simulink model "blackbanana_kinlam_ver2"  (R2022b)
settings: Solver=VariableStepAuto  StartTime=0.0  StopTime=20  RelTol=1e-3
model workspace: external: MAT-File params.mat (data not in the file)
undefined symbols (not defined in the file): cache_size, fleet_size, lambda_allocated_memory, lambda_parallel_instances, message_size, simulation_time, time
libraries: simulink x2, VACLib x1
settings Model: Creator=KarlO  LastModifiedBy=KarlO

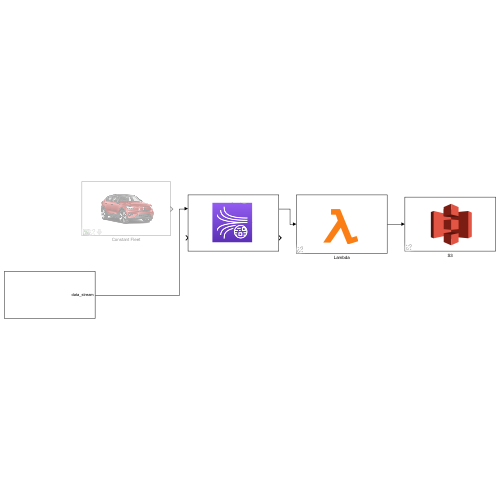
[thumbnail: Simulink's stored preview of the top-level diagram]
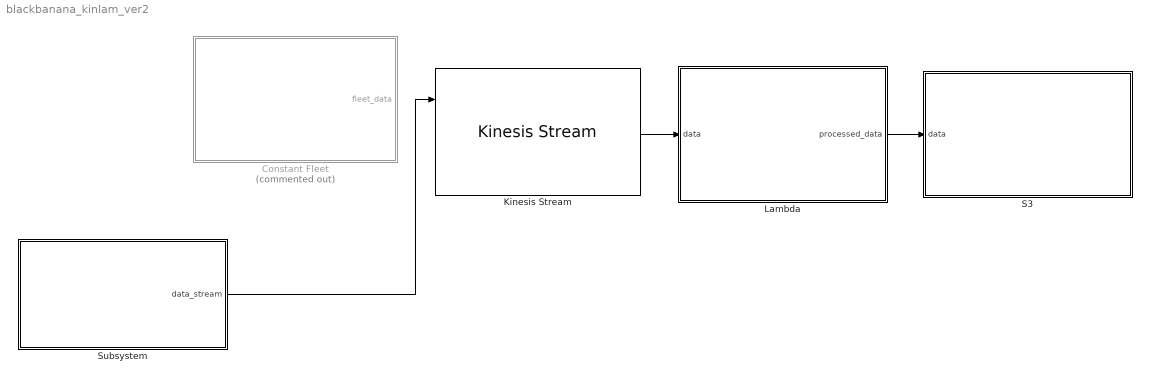
== system blackbanana_kinlam_ver2 ==
  Constant Fleet : Subsystem  Commented=on  AncestorBlock=VACLib/Vehicle Components/Constant Fleet  mask{fleet_size=0, cache_size=0, simulation_time=0, message_size=0}
      settings: LibrarySourceBlock=VACLib/Vehicle Components/Constant Fleet
      mask Display: image('C:\Users\KarlO\architectural-tradeoff-analysis\DCA-simulator\Volvo Architecture\VAC library\Images\VAC\cc9459c7a9e4acd4eb37509497aa20bf.png',[40,10,125,100]); % Use "Edit Image" on toolstrip to change.
  Kinesis Stream : VACLib/AWS Components/Kinesis Stream  SystemSampleTime=-1  VariantActivationTime=update diagram  Latency=0  AutoFrameSizeCalculation=off
      settings: SourceProductName=Volvo Architechture Components
  Lambda : Subsystem  AncestorBlock=VACLib/AWS Components/Lambda
      settings: LibrarySourceBlock=VACLib/AWS Components/Lambda
      mask Display: image('C:\Users\KarlO\architectural-tradeoff-analysis\DCA-simulator\Volvo Architecture\VAC library\Images\VAC\aws-lambda-1.svg',[60,20,80,80]); % Use "Edit Image" on toolstrip to change.
  S3 : Subsystem  AncestorBlock=VACLib/AWS Components/S3
      settings: LibrarySourceBlock=VACLib/AWS Components/S3
      mask Display: image('C:\Users\KarlO\architectural-tradeoff-analysis\DCA-simulator\Volvo Architecture\VAC library\Images\VAC\Amazon-S3-Logo.svg',[55,10,100,100]); % Use "Edit Image" on toolstrip to change.
  Subsystem : Subsystem
  wires:
  Kinesis Stream/1 -> Lambda/1(data)
  Lambda/1(processed_data) -> S3/1(data)
  Subsystem/1(data_stream) -> Kinesis Stream/1

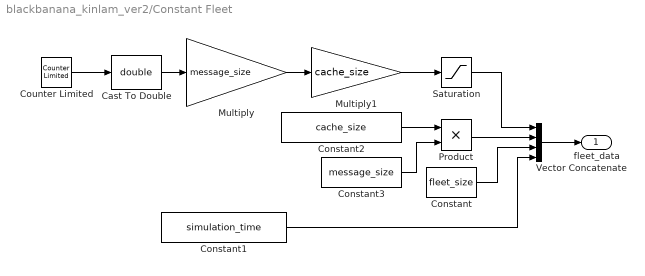
== system blackbanana_kinlam_ver2/Constant Fleet ==
  Cast To Double : DataTypeConversion  OutDataTypeStr=double  SaturateOnIntegerOverflow=off  RndMeth=Floor
  Constant : Constant  Value=fleet_size
  Constant1 : Constant  Value=simulation_time
  Constant2 : Constant  Value=cache_size
  Constant3 : Constant  Value=message_size
  Counter Limited : simulink/Sources/Counter Limited  uplimit=10000000000000  tsamp=(cache_size*message_size)/(fleet_size*message_size)
  Multiply : Gain  Gain=message_size
  Multiply1 : Gain  Gain=cache_size
  Product : Product
  Saturation : Saturate  UpperLimit=fleet_size*time*message_size  LowerLimit=0
  Vector Concatenate : Concatenate  NumInputs=4
  fleet_data : Outport
  wires:
  Vector Concatenate/1 -> fleet_data/1
  Constant/1 -> Vector Concatenate/3
  Constant3/1 -> Product/2
  Product/1 -> Vector Concatenate/2
  Multiply1/1 -> Saturation/1
  Saturation/1 -> Vector Concatenate/1
  Multiply/1 -> Multiply1/1
  Constant2/1 -> Product/1
  Cast To Double/1 -> Multiply/1
  Counter Limited/1 -> Cast To Double/1
  Constant1/1 -> Vector Concatenate/4

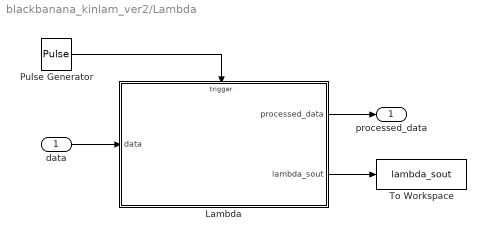
== system blackbanana_kinlam_ver2/Lambda ==
  data : Inport
  Lambda : MATLAB Function  TreatAsAtomicUnit=on
  Pulse Generator : DiscretePulseGenerator  PulseType=Time based  Period=1/log10(lambda_allocated_memory)  PulseWidth=5
  To Workspace : ToWorkspace  VariableName=lambda_sout  SaveFormat=Timeseries  SampleTime=-1
  processed_data : Outport
  wires:
  Lambda/1(processed_data) -> processed_data/1
  Lambda/2(lambda_sout) -> To Workspace/1
  data/1 -> Lambda/1(data)
  Pulse Generator/1 -> Lambda/Trigger

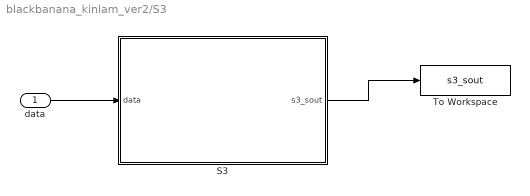
== system blackbanana_kinlam_ver2/S3 ==
  data : Inport
  S3 : MATLAB Function  TreatAsAtomicUnit=on
  To Workspace : ToWorkspace  VariableName=s3_sout  SaveFormat=Timeseries  SampleTime=-1
  wires:
  data/1 -> S3/1(data)
  S3/1(s3_sout) -> To Workspace/1

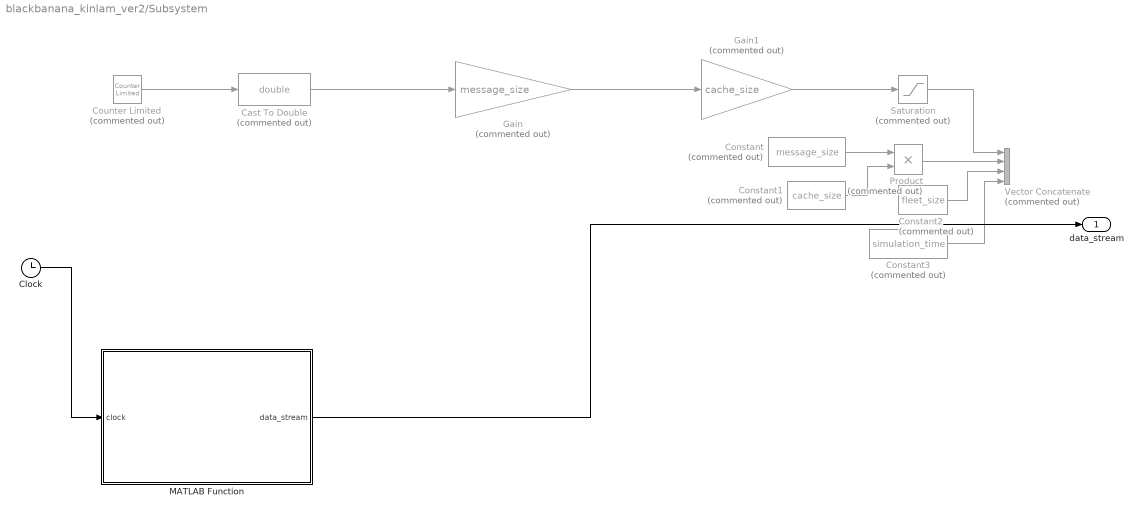
== system blackbanana_kinlam_ver2/Subsystem ==
  Cast To Double : DataTypeConversion  Commented=on  OutDataTypeStr=double  SaturateOnIntegerOverflow=off  RndMeth=Floor
  Clock : Clock
  Constant : Constant  Commented=on  Value=message_size
  Constant1 : Constant  Commented=on  Value=cache_size
  Constant2 : Constant  Commented=on  Value=fleet_size
  Constant3 : Constant  Commented=on  Value=simulation_time
  Counter Limited : simulink/Sources/Counter Limited  Commented=on  uplimit=10000000000000  tsamp=(cache_size*message_size)/(fleet_size*message_size)
  Gain : Gain  Commented=on  Gain=message_size
  Gain1 : Gain  Commented=on  Gain=cache_size
  MATLAB Function : MATLAB Function  TreatAsAtomicUnit=on
  Product : Product  Commented=on
  Saturation : Saturate  Commented=on  LowerLimit=0
  Vector Concatenate : Concatenate  Commented=on  NumInputs=4
  data_stream : Outport
  wires:
  Constant/1 -> Product/1
  Constant1/1 -> Product/2
  Cast To Double/1 -> Gain/1
  Gain1/1 -> Saturation/1
  Counter Limited/1 -> Cast To Double/1
  Product/1 -> Vector Concatenate/2
  Saturation/1 -> Vector Concatenate/1
  Gain/1 -> Gain1/1
  Constant2/1 -> Vector Concatenate/3
  Constant3/1 -> Vector Concatenate/4
  Clock/1 -> MATLAB Function/1(clock)
  MATLAB Function/1(data_stream) -> data_stream/1

== matlab function blackbanana_kinlam_ver2/Subsystem/MATLAB Function ==
  data: clock input; data_stream output; message_size parameter; cache_size parameter; simulation_time parameter; fleet_size parameter
function data_stream  = fcn(clock, message_size, cache_size, simulation_time, fleet_size)

persistent out;
persistent last_tick;
persistent data_to_send;

if isempty(out)
    out = 0;
    data_to_send = (message_size*fleet_size*simulation_time);
    last_tick = 0;
end

tick = clock;
passed_time = tick-last_tick;
last_tick = tick;

send_this_tick = (data_to_send/simulation_time)*passed_time;

to_send = floor(send_this_tick/(cache_size*message_size));

if tick >= simulation_time
    out = data_to_send;
else
    out = out + (to_send*cache_size*message_size);
end

data_stream = [out,(cache_size*message_size), fleet_size, simulation_time];

== matlab function blackbanana_kinlam_ver2/Lambda/Lambda ==
  data: processed_data output; data input; lambda_sout output; lambda_parallel_instances parameter; lambda_allocated_memory parameter
  events: clock input RISING_EDGE_EVENT
function [processed_data,lambda_sout]= lambda(data, lambda_parallel_instances, lambda_allocated_memory)
%Price of lambda instance depends on memory allocated to it
%An increase in memory size triggers an equivalent increase in CPU available to your function.

% Data left in lambda queue to process
persistent remaining_data;
% Chunk size on incoming data
persistent chunk_size;
% Previously received to detect change in incoming data
persistent prev_received;

% Output variables
persistent lambda_cost;
persistent lambda_latency;

%Limited for 1 to be divisible by computation time 1/x = even
computation_time = 1/log10(lambda_allocated_memory);

if isempty(remaining_data)
    remaining_data = 0;
    prev_received = 0;
    lambda_latency = 0;
    lambda_cost = 0;
end

% Get new data - 0 if no change
new_data = max(0,data(1) - prev_received);
prev_received = prev_received + new_data;
remaining_data = remaining_data + new_data;
chunk_size = data(2);

chunks_to_process = floor(lambda_allocated_memory / chunk_size);
effective_size_processed = (chunks_to_process*chunk_size);

% How many lambda computations is left on currently remaining data
computations_left = remaining_data / effective_size_processed;

if remaining_data > 0
    % Get max number of possible computations if computations left is
    % higher than what can be done in one go 
    computations = min(lambda_parallel_instances,computations_left);

    % Subtract data to be processed
    remaining_data = remaining_data - (computations * effective_size_processed);

    % Calculate memory size needed for lambda
    allocated_memory = lambda_allocated_memory;

    % Calculate lambda pricing

    % GB capacity in parallel
    configured_concurr = lambda_parallel_instances*(allocated_memory/1000);
    % GB seconds used
    provisioned_concurr = configured_concurr * 0.2;
    % $0.0000041667 per GBs
    concurr_cost = provisioned_concurr * 0.0000041667;
    % $0.2 per 1M requests
    request_cost = (computations/1000000) * 0.2;

    % Record cost
    lambda_cost = lambda_cost + concurr_cost + request_cost;

    if remaining_data > 0 
        lambda_latency = max(lambda_latency, (remaining_data/(effective_size_processed*computations))*computation_time);
    end
end

processed_data = [prev_received-remaining_data, data(2), data(3), data(4)];
lambda_sout = [lambda_latency, lambda_cost, 0,0];

== matlab function blackbanana_kinlam_ver2/S3/S3 ==
  data: data input; s3_sout output
function s3_sout = S3(data)

% Keeps count of amount of data buckets (MB)
persistent in_storage;
% Overall cost for usage
persistent s3_cost;

if isempty(in_storage)
    in_storage = 0;
    s3_cost = 0;
end

% Received data (Might be zero if read in between pulses)
% data_packets = (size_sent_in_total, size_of_each_file)
new_data = max(0,data(1) - in_storage);
in_storage = in_storage + new_data;
chunk_size = data(2);

if (new_data > 0)
    % Count packets
    no_of_packets = chunk_size/new_data;
    % Upfront cost ($0.005 per 1000 PUT)
    s3_cost = s3_cost + no_of_packets*0.000005;
end

% [latency, cost, reliability, scalability]
s3_sout = [0, s3_cost,0,0];
